simulink model "hardwareModel_6"  (R2020a)
settings: Solver=FixedStepAuto  StartTime=0.0  StopTime=inf  RelTol=1e-3  EnableMultiTasking=on
values from neighbouring files (symbols this model uses):
  Ts = 0.01    [modelParameters.m]
libraries: mkrmotorcarrierlib x3, simulink x1, eeGeneralControl x1, arduinosensorlib x1
settings Model: SILPILModeSetting=veronly  ExtModeTrigDuration=2  Creator=bkhusain  LastModifiedBy=mmarathe
settings OptimizationCC: EnhancedBackFolding=on  PassReuseOutputArgsAs=Individual arguments  ZeroExternalMemoryAtStartup=off  ZeroInternalMemoryAtStartup=off  MaxStackSize=64  OptimizeBlockOrder=speed  DifferentSizesBufferReuse=on  OptimizationCustomize=off  EfficientTunableParamExpr=on
settings DebuggingCC: ParameterTunabilityLossMsg=error
settings HardwareCC: ProdBitPerPointer=32  ProdBitPerSizeT=32  ProdBitPerPtrDiffT=32  ProdLargestAtomicInteger=Long  ProdLargestAtomicFloat=Double  ProdWordSize=32  ProdHWDeviceType=ARM Compatible->ARM Cortex  UseEmbeddedCoderFeatures=off  UseSimulinkCoderFeatures=off
settings SFSimCC: MATLABDynamicMemAlloc=off
settings RTWCC: SystemTargetFile=ert.tlc  HardwareBoard=Arduino Nano 33 IoT  TLCOptions=-aInlineSetEventsForThisBaseRateFcn=TLC_FALSE -aSuppressMultiTaskScheduler=TLC_FALSE -aRateBasedStepFcn=1  TemplateMakefile=ert_default_tmf  Toolchain=Arduino ARM  BuildConfiguration=Faster Runs
settings CodeAppCC: ForceParamTrailComments=on  IgnoreCustomStorageClasses=off  OperatorAnnotations=on  SimulinkDataObjDesc=on  SFDataObjDesc=on  InsertBlockDesc=on
settings ERTTargetCC: SupportContinuousTime=on  SupportNonInlinedSFcns=on  SupportVariableSizeSignals=on  ExtModeStaticAllocSize=8192

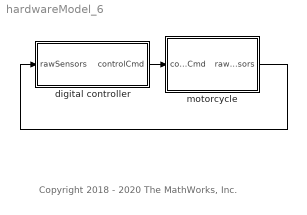
== system hardwareModel_6 ==
  note: Copyright 2018 - 2020 The MathWorks, Inc.
  digital controller : Subsystem
      mask Display: image('$imagefile'); % Use "Edit Image" on toolstrip to change.
  motorcycle : Subsystem
      mask Display: image('$imagefile'); % Use "Edit Image" on toolstrip to change.
  wires:
  digital controller/1(controlCmd) -> motorcycle/1(controlCmd)
  motorcycle/1(rawSensors) -> digital controller/1(rawSensors)

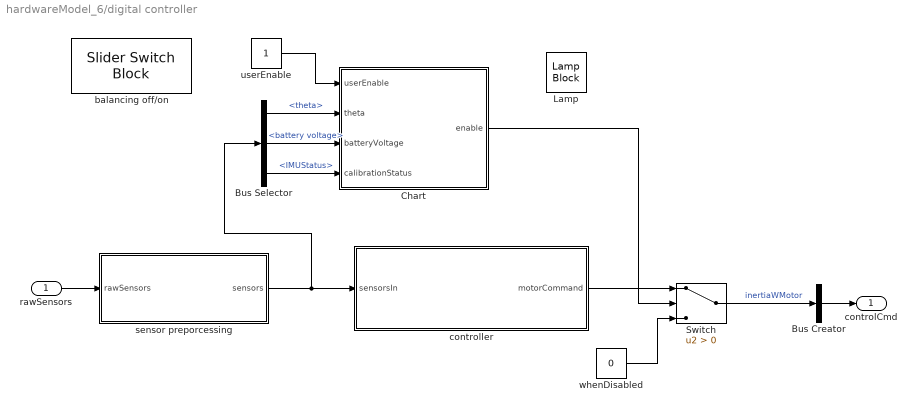
== system hardwareModel_6/digital controller ==
  rawSensors : Inport
  Bus Creator : BusCreator  Inputs=1
  Bus Selector : BusSelector  OutputSignals=theta,battery voltage,IMUStatus
  Chart : Stateflow chart  TreatAsAtomicUnit=on
  Lamp : LampBlock
  Switch : Switch  Criteria=u2 > Threshold
  balancing off/on : SliderSwitchBlock  LabelPosition=Hide
      settings: Values={{'Off', 'On'}, [0 1]}
  controller : Subsystem
  sensor preporcessing : Subsystem
  userEnable : Constant  SampleTime=Ts
  whenDisabled : Constant  Value=0  SampleTime=Ts
  controlCmd : Outport
  wires:
  Switch/1 -> Bus Creator/1  "inertiaWMotor"
  Bus Creator/1 -> controlCmd/1
  rawSensors/1 -> sensor preporcessing/1(rawSensors)
  sensor preporcessing/1(sensors) -> controller/1(sensorsIn), Bus Selector/1
  whenDisabled/1 -> Switch/3
  Chart/1(enable) -> Switch/2
  Bus Selector/1 -> Chart/2(theta)  "<theta>"
  Bus Selector/2 -> Chart/3(batteryVoltage)  "<battery voltage>"
  Bus Selector/3 -> Chart/4(calibrationStatus)  "<IMUStatus>"
  userEnable/1 -> Chart/1(userEnable)
  controller/1(motorCommand) -> Switch/1

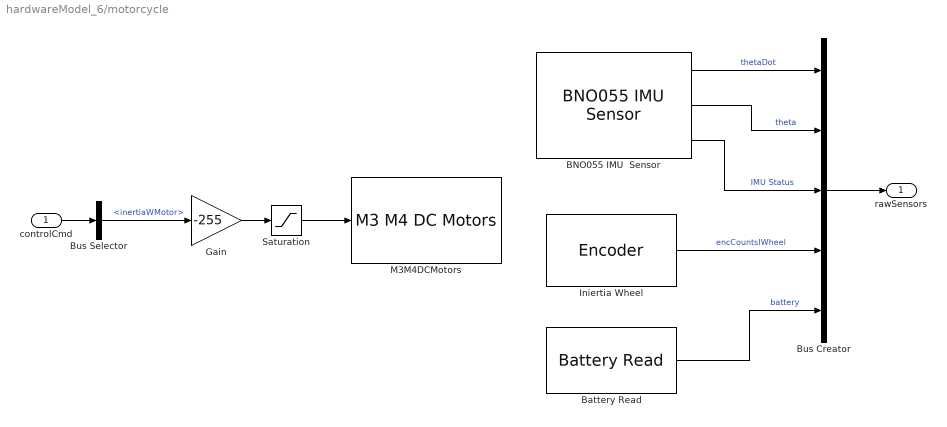
== system hardwareModel_6/motorcycle ==
  controlCmd : Inport
  BNO055 IMU  Sensor : arduinosensorlib/BNO055 IMU Sensor  SlaveAddress=0x28  OperationMode=Fusion  Accel=off  AngularRate=on  MagField=off  EulerAngles=on  Quat=off  LinearAccel=off  GravityVector=off  AccelRange=4G  AccelBW=62.5 Hz  GyroRange=2000 dps  GyroBW=32 Hz  MagODR=10 Hz  SampleTime=Ts  blockPlatform=ARDUINO
      settings: SourceProductName=Simulink Support for Arduino Sensors
  Battery Read : mkrmotorcarrierlib/Battery Read  SlaveAddress=uint8( hex2dec( '66' ) )  blockPlatform=ARDUINO  SampleTime=Ts
      settings: SourceProductName=Simulink Support for Arduino MKR Motor Shield
  Bus Creator : BusCreator  Inputs=5
  Bus Selector : BusSelector  OutputSignals=inertiaWMotor
  Gain : Gain  Gain=-255
  Iniertia Wheel : mkrmotorcarrierlib/Encoder  SlaveAddress=uint8( hex2dec( '66' ) )  blockPlatform=ARDUINO  Encoder=1  ShowSpeed=off  ResetOption=on  SampleTime=Ts
      settings: SourceProductName=Simulink Support for Arduino MKR Motor Carrier
  M3M4DCMotors : mkrmotorcarrierlib/M3 M4 DC Motors  MotorNumber=M3  forwardPinNumber=2  reversePinNumber=3
      settings: SourceProductName=Simulink Support for Arduino MKR Motor Carrier
  Saturation : Saturate  UpperLimit=255  LowerLimit=-255
  rawSensors : Outport
  wires:
  BNO055 IMU  Sensor/1 -> Bus Creator/1  "thetaDot"
  BNO055 IMU  Sensor/2 -> Bus Creator/2  "theta"
  BNO055 IMU  Sensor/3 -> Bus Creator/3  "IMU Status"
  Iniertia Wheel/1 -> Bus Creator/4  "encCountsIWheel"
  Battery Read/1 -> Bus Creator/5  "battery"
  Bus Creator/1 -> rawSensors/1
  controlCmd/1 -> Bus Selector/1
  Gain/1 -> Saturation/1
  Bus Selector/1 -> Gain/1  "<inertiaWMotor>"
  Saturation/1 -> M3M4DCMotors/1

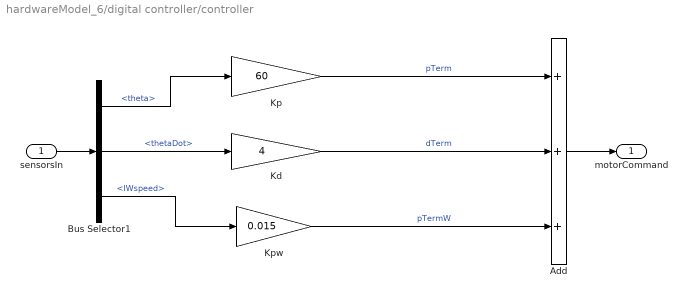
== system hardwareModel_6/digital controller/controller ==
  sensorsIn : Inport
  Add : Sum  Inputs=+++
  Bus Selector1 : BusSelector  OutputSignals=theta,thetaDot,IWspeed
  Kd : Gain  Gain=4
  Kp : Gain  Gain=60
  Kpw : Gain  Gain=0.015
  motorCommand : Outport
  wires:
  Bus Selector1/3 -> Kpw/1  "<IWspeed>"
  Kpw/1 -> Add/3  "pTermW"
  Kd/1 -> Add/2  "dTerm"
  Bus Selector1/2 -> Kd/1  "<thetaDot>"
  Bus Selector1/1 -> Kp/1  "<theta>"
  Kp/1 -> Add/1  "pTerm"
  sensorsIn/1 -> Bus Selector1/1
  Add/1 -> motorCommand/1

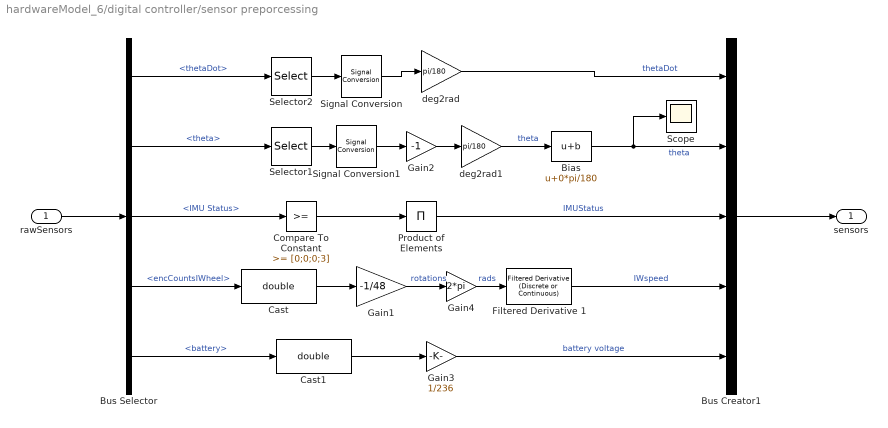
== system hardwareModel_6/digital controller/sensor preporcessing ==
  rawSensors : Inport
  Bias : Bias  Bias=0*pi/180
  Bus Creator1 : BusCreator  Inputs=5
  Bus Selector : BusSelector  OutputSignals=thetaDot,theta,IMU Status,encCountsIWheel,battery
  Cast : DataTypeConversion  OutDataTypeStr=double
  Cast1 : DataTypeConversion  OutDataTypeStr=double
  Compare To Constant : simulink/Logic and Bit Operations/Compare To Constant  relop=>=  const=[0;0;0;3]  OutDataTypeStr=boolean
  Filtered Derivative 1 : eeGeneralControl/Filtered Derivative (Discrete or Continuous)  K=1  T=0.1  B=inf  A=-inf  minRatio=10  init_option=Inherited from block input  x0=0  Ts=Ts
      settings: SourceProductBaseCode=PS
  Gain1 : Gain  Gain=-1/48
  Gain2 : Gain  Gain=-1
  Gain3 : Gain  Gain=1/236
  Gain4 : Gain  Gain=2*pi
  Product of Elements : Product  Inputs=*
  Scope : Scope
  Selector1 : Selector  InputPortWidth=3  IndexOptions=Index vector (dialog)  Indices=[2]  OutputSizes=1
  Selector2 : Selector  InputPortWidth=3  IndexOptions=Index vector (dialog)  Indices=[2]  OutputSizes=1
  Signal Conversion : SignalConversion  OverrideOpt=off
  Signal Conversion1 : SignalConversion  OverrideOpt=off
  deg2rad : Gain  Gain=pi/180
  deg2rad1 : Gain  Gain=pi/180
  sensors : Outport
  wires:
  Bus Selector/4 -> Cast/1  "<encCountsIWheel>"
  Compare To Constant/1 -> Product of Elements/1
  Bus Selector/5 -> Cast1/1  "<battery>"
  Selector2/1 -> Signal Conversion/1
  Bus Selector/2 -> Selector1/1  "<theta>"
  Selector1/1 -> Signal Conversion1/1
  Cast1/1 -> Gain3/1
  Bus Selector/3 -> Compare To Constant/1  "<IMU Status>"
  rawSensors/1 -> Bus Selector/1
  Product of Elements/1 -> Bus Creator1/3  "IMUStatus"
  Filtered Derivative 1/1 -> Bus Creator1/4  "IWspeed"
  deg2rad1/1 -> Bias/1  "theta"
  Bus Selector/1 -> Selector2/1  "<thetaDot>"
  Gain3/1 -> Bus Creator1/5  "battery voltage"
  Bus Creator1/1 -> sensors/1
  Signal Conversion1/1 -> Gain2/1
  Gain2/1 -> deg2rad1/1
  Signal Conversion/1 -> deg2rad/1
  Cast/1 -> Gain1/1
  Gain1/1 -> Gain4/1  "rotations"
  Gain4/1 -> Filtered Derivative 1/1  "rads"
  deg2rad/1 -> Bus Creator1/1  "thetaDot"
  Bias/1 -> Scope/1, Bus Creator1/2  "theta"

== stateflow chart hardwareModel_6/digital controller/Chart ==
  state checkFallen [parallel]
    settings: executionOrder=1
    state fallen
      entry: upright = false
    state standing
      entry: upright = true
    (default) -> fallen
    fallen -> standing : [abs(theta) <pi*12/180]
    standing -> fallen : [abs(theta) > pi*12/180]
  state checkIMUCalib [parallel]
    settings: executionOrder=2
    state imuNotCalibrated
      entry:
      IMUCalibrated = false;
    state imuCalibrated
      entry:
      IMUCalibrated = true;
    (default) -> imuNotCalibrated
    imuNotCalibrated -> imuCalibrated : [calibrationStatus == true]
  state checkBattery [parallel]
    settings: executionOrder=3
    state batteryNotCharged
      entry:
      batteryOK = false;
    state batteryCharged
      entry:
      batteryOK = true;
    (default) -> batteryNotCharged
    batteryCharged -> batteryNotCharged : [batteryVoltage < 3.0]
    batteryNotCharged -> batteryCharged : [batteryVoltage >= 3.0]
  state calculateEnable [parallel]
    settings: executionOrder=4
    state disableControl
      entry: enable = false
    state enableControl
      entry: enable = true
    (default) -> disableControl
    disableControl -> enableControl : [userEnable&& batteryOK && IMUCalibrated && upright]
    enableControl -> disableControl : [not(userEnable) || not(batteryOK) || not(IMUCalibrated) || not(upright)]
  data: userEnable input; theta input; enable output; batteryVoltage input; calibrationStatus input; upright local; IMUCalibrated local; batteryOK local
